simulink model "pend_lqr"  (Simulink 9.1)
settings: Solver=ode4  StartTime=0.0  StopTime=20  FixedStep=0.01  RelTol=1e-3  EnableMultiTasking=on
values from neighbouring files (symbols this model uses):
  K = lqr(As,Bs,Q,R)    [pend_state_estimator_init.m]
undefined symbols (not defined in the file or in its folder): a, b, c, c2, d, f, h
settings Model: Creator=User  LastModifiedBy=DELL
settings DataIOCC: LimitDataPoints=on  SignalLoggingSaveFormat=ModelDataLogs
settings OptimizationCC: ExpressionDepthLimit=2147483647
settings DebuggingCC: SolverPrmCheckMsg=warning  FcnCallInpInsideContextMsg=warning  StateNameClashWarn=warning
settings GRTTargetCC: GeneratePreprocessorConditionals=Disable all

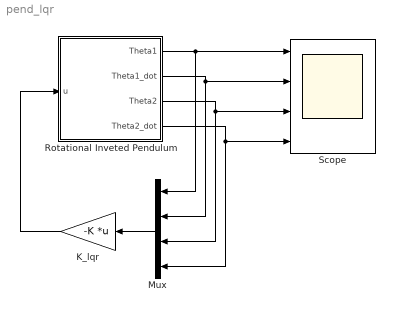
== system pend_lqr ==
  K_lqr : Gain  Gain=-K  Multiplication=Matrix(K*u)
  Mux : Mux
  Rotational Inveted Pendulum : Subsystem
  Scope : Scope  NumInputPorts=4
  wires:
  Rotational Inveted Pendulum/1(Theta1) -> Scope/1, Mux/1
  Rotational Inveted Pendulum/2(Theta1_dot) -> Scope/2, Mux/2
  Rotational Inveted Pendulum/3(Theta2) -> Scope/3, Mux/3
  Rotational Inveted Pendulum/4(Theta2_dot) -> Scope/4, Mux/4
  Mux/1 -> K_lqr/1
  K_lqr/1 -> Rotational Inveted Pendulum/1(u)

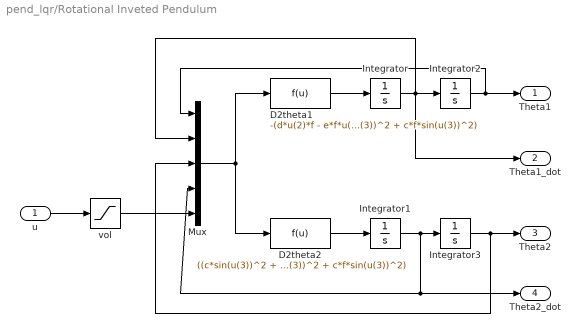
== system pend_lqr/Rotational Inveted Pendulum ==
  u : Inport
  D2theta1 : Fcn  Expr=-(d*u(2)*f - e*f*u(5) + b*c2*u(4)*cos(u(3)) + b*u(4)^2*f*sin(u(3)) - b*h*cos(u(3))*sin(u(3)) - b*c*u(2)^2*cos(u(3))^2*sin(u(3)) + 2*c*u(2)*u(4)*f*cos(u(3))*sin(u(3)))/(a*f - b^2*cos(u(3))^2 + c*f*sin(u(3))^2)
  D2theta2 : Fcn  Expr=((c*sin(u(3))^2 + a)*((c*sin(2*u(3))*u(2)^2)/2 - c2*u(4) + h*sin(u(3))))/(a*f - b^2*cos(u(3))^2 + c*f*sin(u(3))^2) - (b*cos(u(3))*(b*sin(u(3))*u(4)^2 + c*u(2)*sin(2*u(3))*u(4) + d*u(2) - e*u(5)))/(a*f - b^2*cos(u(3))^2 + c*f*sin(u(3))^2)
  Integrator : Integrator
  Integrator1 : Integrator
  Integrator2 : Integrator
  Integrator3 : Integrator  InitialCondition=pi/18
  Mux : Mux  Inputs=5
  vol : Saturate  UpperLimit=25  LowerLimit=-25
  Theta1 : Outport
  Theta1_dot : Outport  Port=2
  Theta2 : Outport  Port=3
  Theta2_dot : Outport  Port=4
  wires:
  u/1 -> vol/1
  Integrator2/1 -> Theta1/1, Mux/1
  Mux/1 -> D2theta1/1, D2theta2/1
  vol/1 -> Mux/5
  D2theta1/1 -> Integrator/1
  Integrator/1 -> Integrator2/1, Theta1_dot/1, Mux/2
  D2theta2/1 -> Integrator1/1
  Integrator1/1 -> Integrator3/1, Theta2_dot/1, Mux/4
  Integrator3/1 -> Theta2/1, Mux/3
